simulink model "duplointegrador_com_obs"  (R2020b)
settings: Solver=ode4  StartTime=0.0  StopTime=10  FixedStep=1e-3  RelTol=1e-3
values from neighbouring files (symbols this model uses):
  h = 0.1    [duplointegrador_script.m]
  x10 = 0    [duplointegrador_script.m]
  x20 = 10    [duplointegrador_script.m]
undefined symbols (not defined in the file or in its folder): Flqr
libraries: eeLuenbergerObserver x1
settings Model: Creator=Trevor  LastModifiedBy=lucas
settings SolverCC: AutoInsertRateTranBlk=on
settings DataIOCC: LimitDataPoints=on  SaveFormat=Array  ReturnWorkspaceOutputs=off
settings OptimizationCC: LifeSpan=inf
settings DebuggingCC: SFUnexpectedBacktrackingDiag=warning  SFNoUnconditionalDefaultTransitionDiag=warning  SFExecutionAtInitializationDiag=none  ArithmeticOperatorsInVariantConditions=warning
settings HardwareCC: ProdBitPerPointer=32  ProdBitPerSizeT=32  ProdBitPerPtrDiffT=32  ProdLargestAtomicFloat=None  ProdIntDivRoundTo=Undefined  ProdEndianess=Unspecified  ProdWordSize=32  ProdHWDeviceType=32-bit Generic
settings ModelReferenceCC: PropagateSignalLabelsOutOfModel=off
settings SFSimCC: SimUseLocalCustomCode=off  CustomCodeUndefinedFunction=UseInterfaceOnly
settings RTWCC: RTWUseLocalCustomCode=off
settings CodeAppCC: StateflowObjectComments=on
settings GRTTargetCC: TargetLangStandard=C89/C90 (ANSI)
settings ConfigComp: CovMetricSettings=dw  CovSaveCumulativeToWorkspaceVar=on  CovSaveSingleToWorkspaceVar=on  CovExternalEMLEnable=off

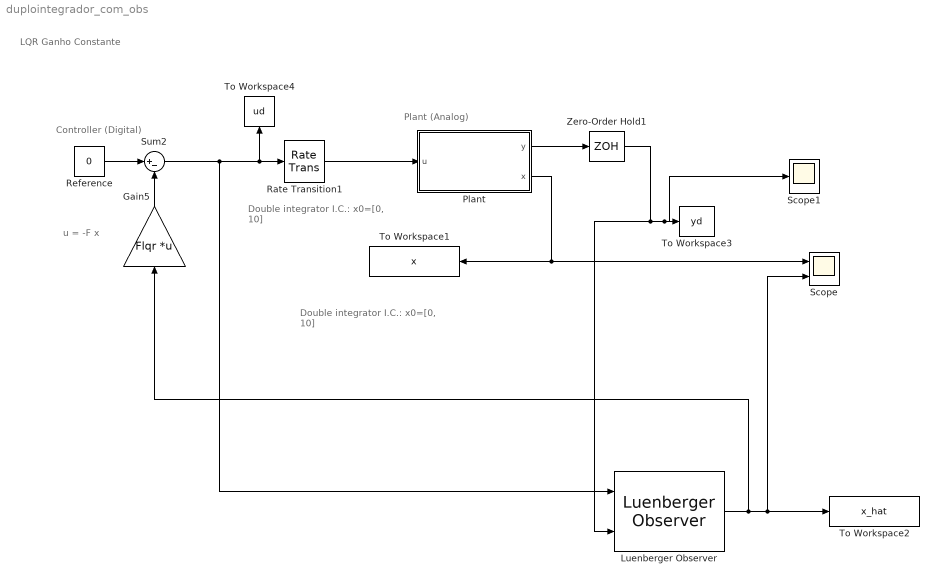
== system duplointegrador_com_obs ==
  note: Double integrator
      | I.C.: x0=[0, 10]
  note: Controller (Digital)
  note: u = -F x
  note: Plant (Analog)
  note: Double integrator
      | I.C.: x0=[0, 10]
  note: LQR Ganho Constante
  Gain5 : Gain  Gain=Flqr  Multiplication=Matrix(K*u) (u vector)
  Luenberger Observer : eeLuenbergerObserver/Luenberger Observer  StateSpaceType=Discrete-time  Ad=Phi  Bd=Gamma  Cd=C  Dd=D  A=1  B=1  C=1  D=1  ObserverDesign=Desired eigenvalues  Ld=1  DesiredEigenvalues=obs_eig  x0=[0;0]  Tsd=0.1  Ts=h
      settings: SourceProductBaseCode=PS
  Plant : Subsystem
      mask Display:
      | text(.5,.6,'dx/dt = Ax + Bu','horizontalAlignment', 'center','verticalAlignment', 'middle','texmode','on')
      | text(.5,.4,'y = Cx + Du','horizontalAlignment', 'center','verticalAlignment', 'middle','texmode','on')
      | port_label('input',1,'u')
      | port_label('output',1,'y')
      | port_label('output',2,'x')
  Rate Transition1 : RateTransition  Integrity=off  OutPortSampleTime=h/10
  Reference : Constant  Value=0  SampleTime=h
  Scope : Scope  NumInputPorts=2
  Scope1 : Scope
  Sum2 : Sum  Inputs=|+-
  To Workspace1 : ToWorkspace  VariableName=x  SaveFormat=Timeseries  SampleTime=h
  To Workspace2 : ToWorkspace  VariableName=x_hat  SaveFormat=Timeseries  SampleTime=h
  To Workspace3 : ToWorkspace  VariableName=yd  SaveFormat=Timeseries  SampleTime=-1
  To Workspace4 : ToWorkspace  VariableName=ud  SaveFormat=Timeseries  SampleTime=h
  Zero-Order Hold1 : ZeroOrderHold  SampleTime=h
  wires:
  Sum2/1 -> To Workspace4/1, Rate Transition1/1, Luenberger Observer/1
  Reference/1 -> Sum2/1
  Plant/1(y) -> Zero-Order Hold1/1
  Plant/2(x) -> Scope/1, To Workspace1/1
  Gain5/1 -> Sum2/2
  Zero-Order Hold1/1 -> Luenberger Observer/2, Scope1/1, To Workspace3/1
  Luenberger Observer/1 -> Scope/2, To Workspace2/1, Gain5/1
  Rate Transition1/1 -> Plant/1(u)

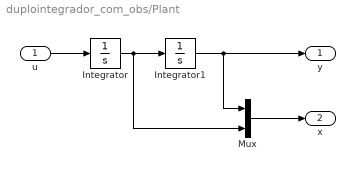
== system duplointegrador_com_obs/Plant ==
  u : Inport
  Integrator : Integrator  InitialCondition=x20
  Integrator1 : Integrator  InitialCondition=x10
  Mux : Mux  Inputs=2
  y : Outport
  x : Outport  Port=2
  wires:
  Integrator/1 -> Mux/2, Integrator1/1
  Integrator1/1 -> y/1, Mux/1
  Mux/1 -> x/1
  u/1 -> Integrator/1
